simulink model "sim1"  (R2015b)
settings: Solver=VariableStepAuto  StartTime=0.0  StopTime=20  RelTol=1e-3
values from neighbouring files (symbols this model uses):
  A1 = [0 1 0 ... (first row only)    [tp2.m]
  A2 = [0 1 0 ... (first row only)    [tp2.m]
  B1 = [0 ... (first row only)    [tp2.m]
  B2 = [0 ... (first row only)    [tp2.m]
settings Model: Creator=max.Sonzogni  LastModifiedBy=max.sonzogni

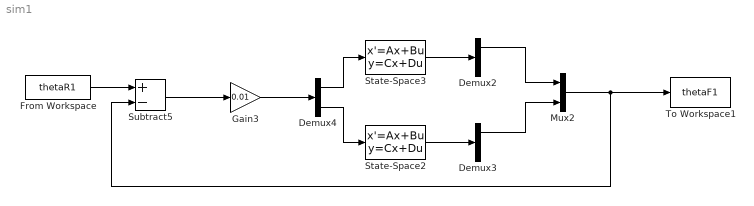
== system sim1 ==
  Demux2 : Demux  Outputs=3
  Demux3 : Demux  Outputs=3
  Demux4 : Demux  Outputs=2
  From Workspace : FromWorkspace  VariableName=thetaR1  SampleTime=0
  Gain3 : Gain  Gain=0.01
  Mux2 : Mux  Inputs=2
  State-Space2 : StateSpace  A=A2  B=B2  C=eye(3)  D=zeros(3,1)  X0=0
  State-Space3 : StateSpace  A=A1  B=B1  C=eye(3)  D=zeros(3,1)  X0=0
  Subtract5 : Sum  Inputs=+-
  To Workspace1 : ToWorkspace  VariableName=thetaF1  SampleTime=-1
  wires:
  State-Space2/1 -> Demux3/1
  State-Space3/1 -> Demux2/1
  Demux2/1 -> Mux2/1
  Demux3/1 -> Mux2/2
  Mux2/1 -> Subtract5/2, To Workspace1/1
  Gain3/1 -> Demux4/1
  Demux4/1 -> State-Space3/1
  Demux4/2 -> State-Space2/1
  From Workspace/1 -> Subtract5/1
  Subtract5/1 -> Gain3/1
